simulink model "Dinamica_longitudinale_leader_ubuntu_param"  (R2020b)
settings: Solver=ode23s  StartTime=0.0  StopTime=100  FixedStep=0.0001
model workspace (MAT data in the model file):
  a1 = Simulink.Parameter
  a1.Value = 2
  a1.DataType = 'auto'
  a1.Dimensions = [1 1]
  a2 = Simulink.Parameter
  a2.Value = 0.5
  a2.DataType = 'auto'
  a2.Dimensions = [1 1]
  a3 = Simulink.Parameter
  a3.Value = -1.5
  a3.DataType = 'auto'
  a3.Dimensions = [1 1]
  a4 = Simulink.Parameter
  a4.Value = 1.2
  a4.DataType = 'auto'
  a4.Dimensions = [1 1]
  a5 = Simulink.Parameter
  a5.Value = -1
  a5.DataType = 'auto'
  a5.Dimensions = [1 1]
  a6 = Simulink.Parameter
  a6.Value = 1
  a6.DataType = 'auto'
  a6.Dimensions = [1 1]
  aero_drag_coeff = Simulink.Parameter
  aero_drag_coeff.Value = 0.3
  aero_drag_coeff.DataType = 'auto'
  aero_drag_coeff.Dimensions = [1 1]
  frontal_area = Simulink.Parameter
  frontal_area.Value = 2
  frontal_area.DataType = 'auto'
  frontal_area.Dimensions = [1 1]
  initialDesiredSpeed = Simulink.Parameter
  initialDesiredSpeed.Value = 0
  initialDesiredSpeed.DataType = 'auto'
  initialDesiredSpeed.Dimensions = [1 1]
  initialPosition = Simulink.Parameter
  initialPosition.Value = 10
  initialPosition.DataType = 'auto'
  initialPosition.Dimensions = [1 1]
  initialRotation = Simulink.Parameter
  initialRotation.Value = 0.001
  initialRotation.DataType = 'auto'
  initialRotation.Dimensions = [1 1]
  initialSpeed = Simulink.Parameter
  initialSpeed.Value = 0.001
  initialSpeed.DataType = 'auto'
  initialSpeed.Dimensions = [1 1]
  k = Simulink.Parameter
  k.Value = 500
  k.DataType = 'auto'
  k.Dimensions = [1 1]
  mass = Simulink.Parameter
  mass.Value = 1350
  mass.DataType = 'auto'
  mass.Dimensions = [1 1]
  maxRotation = Simulink.Parameter
  maxRotation.Value = 1000000
  maxRotation.DataType = 'auto'
  maxRotation.Dimensions = [1 1]
  maxSpeed = Simulink.Parameter
  maxSpeed.Value = 50
  maxSpeed.DataType = 'auto'
  maxSpeed.Dimensions = [1 1]
  minRotation = Simulink.Parameter
  minRotation.Value = -1000000
  minRotation.DataType = 'auto'
  minRotation.Dimensions = [1 1]
  minSpeed = Simulink.Parameter
  minSpeed.Value = -50
  minSpeed.DataType = 'auto'
  minSpeed.Dimensions = [1 1]
  t1 = Simulink.Parameter
  t1.Value = 10
  t1.DataType = 'auto'
  t1.Dimensions = [1 1]
  t1_wet = Simulink.Parameter
  t1_wet.Value = 999
  t1_wet.DataType = 'auto'
  t1_wet.Dimensions = [1 1]
  t2 = Simulink.Parameter
  t2.Value = 20
  t2.DataType = 'auto'
  t2.Dimensions = [1 1]
  t2_snow = Simulink.Parameter
  t2_snow.Value = 999
  t2_snow.DataType = 'auto'
  t2_snow.Dimensions = [1 1]
  t3 = Simulink.Parameter
  t3.Value = 30
  t3.DataType = 'auto'
  t3.Dimensions = [1 1]
  t3_ice = Simulink.Parameter
  t3_ice.Value = 999
  t3_ice.DataType = 'auto'
  t3_ice.Dimensions = [1 1]
  t4 = Simulink.Parameter
  t4.Value = 40
  t4.DataType = 'auto'
  t4.Dimensions = [1 1]
  t5 = Simulink.Parameter
  t5.Value = 50
  t5.DataType = 'auto'
  t5.Dimensions = [1 1]
  v_height = Simulink.Parameter
  v_height.Value = 0.75
  v_height.DataType = 'auto'
  v_height.Dimensions = [1 1]
libraries: simulink x1
settings Model: ParameterArgumentNames=a1,a2,a3,a4,a5,a6,aero_drag_coeff,frontal_area,initialDesiredSpeed,initialPosition,initialRotation,initialSpeed,k,mass,maxRotation,maxSpeed,minRotation,minSpeed,t1,t1_wet,t2,t2_snow,t3,t3_ice,t4,t5,v_height  OrderedModelArguments=off  Creator=salvo  LastModifiedBy=ubuntu

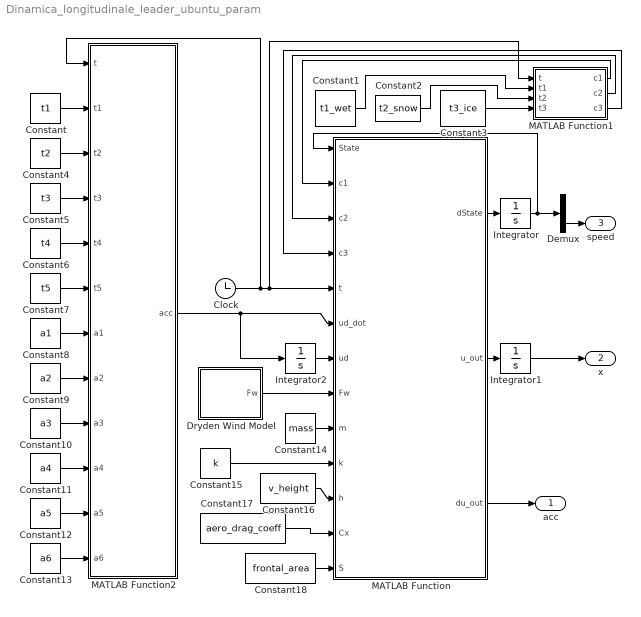
== system Dinamica_longitudinale_leader_ubuntu_param ==
  Clock : Clock
  Constant : Constant  Value=t1
  Constant1 : Constant  Value=t1_wet
  Constant10 : Constant  Value=a3
  Constant11 : Constant  Value=a4
  Constant12 : Constant  Value=a5
  Constant13 : Constant  Value=a6
  Constant14 : Constant  Value=mass
  Constant15 : Constant  Value=k
  Constant16 : Constant  Value=v_height
  Constant17 : Constant  Value=aero_drag_coeff
  Constant18 : Constant  Value=frontal_area
  Constant2 : Constant  Value=t2_snow
  Constant3 : Constant  Value=t3_ice
  Constant4 : Constant  Value=t2
  Constant5 : Constant  Value=t3
  Constant6 : Constant  Value=t4
  Constant7 : Constant  Value=t5
  Constant8 : Constant  Value=a1
  Constant9 : Constant  Value=a2
  Demux : Demux  Outputs=2
  Dryden Wind Model : Subsystem
  Integrator : Integrator  InitialCondition=[initialRotation;initialSpeed]  LimitOutput=on  UpperSaturationLimit=[maxRotation;maxSpeed]  LowerSaturationLimit=[minRotation;minSpeed]
  Integrator1 : Integrator  InitialCondition=initialPosition
  Integrator2 : Integrator  InitialCondition=initialDesiredSpeed  LimitOutput=on  UpperSaturationLimit=maxSpeed  LowerSaturationLimit=minSpeed
  MATLAB Function : MATLAB Function  TreatAsAtomicUnit=on
  MATLAB Function1 : MATLAB Function  TreatAsAtomicUnit=on
  MATLAB Function2 : MATLAB Function  TreatAsAtomicUnit=on
  acc : Outport
  x : Outport  Port=2
  speed : Outport  Port=3
  wires:
  MATLAB Function/1(dState) -> Integrator/1
  Integrator/1 -> Demux/1, MATLAB Function/1(State)
  Clock/1 -> MATLAB Function2/1(t), MATLAB Function1/1(t), MATLAB Function/5(t)
  MATLAB Function2/1(acc) -> MATLAB Function/6(ud_dot), Integrator2/1
  MATLAB Function/2(u_out) -> Integrator1/1
  Integrator1/1 -> x/1
  Integrator2/1 -> MATLAB Function/7(ud)
  MATLAB Function1/3(c3) -> MATLAB Function/4(c3)
  MATLAB Function1/2(c2) -> MATLAB Function/3(c2)
  MATLAB Function1/1(c1) -> MATLAB Function/2(c1)
  MATLAB Function/3(du_out) -> acc/1
  Dryden Wind Model/1(Fw) -> MATLAB Function/8(Fw)
  Demux/2 -> speed/1
  Constant1/1 -> MATLAB Function1/2(t1)
  Constant2/1 -> MATLAB Function1/3(t2)
  Constant3/1 -> MATLAB Function1/4(t3)
  Constant/1 -> MATLAB Function2/2(t1)
  Constant4/1 -> MATLAB Function2/3(t2)
  Constant5/1 -> MATLAB Function2/4(t3)
  Constant13/1 -> MATLAB Function2/12(a6)
  Constant12/1 -> MATLAB Function2/11(a5)
  Constant11/1 -> MATLAB Function2/10(a4)
  Constant6/1 -> MATLAB Function2/5(t4)
  Constant7/1 -> MATLAB Function2/6(t5)
  Constant8/1 -> MATLAB Function2/7(a1)
  Constant9/1 -> MATLAB Function2/8(a2)
  Constant10/1 -> MATLAB Function2/9(a3)
  Constant14/1 -> MATLAB Function/9(m)
  Constant15/1 -> MATLAB Function/10(k)
  Constant16/1 -> MATLAB Function/11(h)
  Constant17/1 -> MATLAB Function/12(Cx)
  Constant18/1 -> MATLAB Function/13(S)

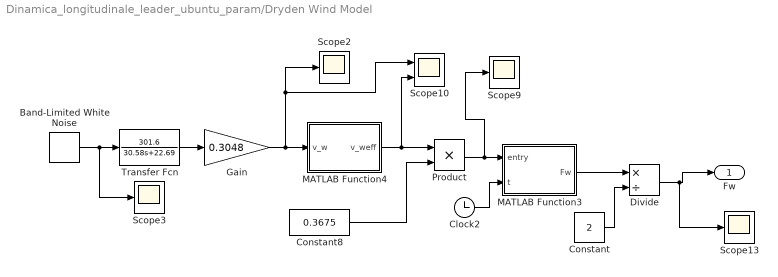
== system Dinamica_longitudinale_leader_ubuntu_param/Dryden Wind Model ==
  Band-Limited White Noise : simulink/Sources/Band-Limited White Noise  Cov=50  Ts=0.1  seed=[23341]
  Clock2 : Clock
  Constant : Constant  Value=2
  Constant8 : Constant  Value=0.3675
  Divide : Product  Inputs=*/
  Gain : Gain  Gain=0.3048
  MATLAB Function3 : MATLAB Function  TreatAsAtomicUnit=on
  MATLAB Function4 : MATLAB Function  TreatAsAtomicUnit=on
  Product : Product
  Scope10 : Scope  NumInputPorts=2
  Scope{2..3,9,13} (4 alike) : Scope
  Transfer Fcn : TransferFcn  Numerator=[301.6]  Denominator=[0 30.58 22.69]
  Fw : Outport  VectorParamsAs1DForOutWhenUnconnected=off
  wires:
  Constant8/1 -> Product/2
  Band-Limited White Noise/1 -> Transfer Fcn/1, Scope3/1
  Product/1 -> Scope9/1, MATLAB Function3/1(entry)
  Clock2/1 -> MATLAB Function3/2(t)
  Gain/1 -> MATLAB Function4/1(v_w), Scope2/1, Scope10/1
  MATLAB Function4/1(v_weff) -> Scope10/2, Product/1
  Transfer Fcn/1 -> Gain/1
  MATLAB Function3/1(Fw) -> Divide/1
  Constant/1 -> Divide/2
  Divide/1 -> Scope13/1, Fw/1

== matlab function Dinamica_longitudinale_leader_ubuntu_param/Dryden Wind Model/MATLAB Function4 ==
  data: v_w input; v_weff output
function v_weff = fcn(v_w)

v_wquadro = (v_w)^2;

if v_w >=0
    v_weff = v_wquadro;
else
    v_weff = -v_wquadro;
end

== matlab function Dinamica_longitudinale_leader_ubuntu_param/MATLAB Function ==
  data: State input; c1 input; c2 input; c3 input; t input; ud_dot input; dState output; ud input; Fw input; u_out output; du_out output; m input; k input; h input; Cx input; S input
function [dState, u_out, du_out] = long_dyn(State, c1, c2, c3, t, ud_dot, ud, Fw, m, k, h, Cx, S) 
%c1,c2 e c3 sono i coefficienti di Burckhardt per il calcolo dell'attrito
%ud --> velocità desiderata
%ud_dot --> accelerazione desiderata (derivata di ud)
%Fw --> Forza del vento opposta al senso di marcia

w = State(1);   % rotazione ruota
u = State(2);   % velocità long

%m = 1350; %Massa del veicolo [Kg]

ro = 1.225; %Densità dell'aria [Kg/m^3]
%S = 2; %Superficie bagnata longitudinale [m^2]
%Cx = 0.3; %Coefficiente di resistenza longitudinale 
F_aero = 0.5*ro*S*Cx*u^2; %Forza aerodinamica [N] - formula 4.2 cap.4

%f = 0.01; %Coefficiente di resistenza al rotolamento
g = 9.81; %Accelerazione di gravità [m/s^2]
a1 = 1.51; %Semipasso anteriore [m]
a2 = 1.288; %Semipasso posteriore [m]
l = a1+a2; %Passo [m]

C0 = 9.91*10^-3; %Coefficienti tipici per pneumatici radiali
C1 = 1.95*10^-5;
C2 = 1.76*10^-9;
Rxt = C0+C1*u+C2*u^4; %Resistenza al rotolamento complessiva [N]

%Fattori contrastanti il senso di marcia - formula 4.1. 
%Include Fw che è il vento
FLoss = Fw+Rxt+F_aero;

Iw = 1.125; % momento inerziale della ruota [Kg*m^2]
%h = 0.75; % Altezza del baricentro rispetto al suolo [m]

FzR = m*g*a1/l + m*h*ud_dot/l; %Trasferimento di carico assale posteriore [N]
Fz = FzR; %Carico normale totale agente sulla vettura [N]
kt = 150000; %Rigidezza verticale ruota motrice [N/m]

R_w = 0.5; %Raggio indeformato [m]
R_s = R_w - Fz/kt; %Raggio statico [m]
x = acos(complex(R_s/R_w));
R = real((sin(x)/x)*R_w); %Raggio effettivo [m]

%k = 500;

%calcolo coppia desiderata (eq.28 paper "Pedone")
Tw = (Iw/R)*(ud_dot - k*(u-ud));

if w*R>u
    sigma = (w*R-u)/(w*R); %Slittamento longitudinale in fase di accelerazione 
elseif (w*R)==u
    sigma = 0;
else
    sigma = (w*R-u)/u; %Slittamento longitudinale in fase di frenatura
end

mu = c1*(1-exp(-c2*sigma))-c3*sigma;

% Forza longitudinale delle ruote (Fxf+Fxr)
Fx2 = mu*Fz; 

dw = 1/Iw*(Tw-R*Fx2); %Dinamica rotazionale ruota motrice - (4.38)
du = 1/m*(Fx2-FLoss); %Din Longitudinale - (4.1)

dState = [dw du]';
u_out = u;

if t<0.1
    du_out = 0;
else
    du_out = du;
end

end

== matlab function Dinamica_longitudinale_leader_ubuntu_param/MATLAB Function2 ==
  data: t input; acc output; t1 input; t2 input; t3 input; t4 input; t5 input; a1 input; a2 input; a3 input; a4 input; a5 input; a6 input
function acc  = driver_acc(t, t1, t2, t3, t4, t5, a1, a2, a3, a4, a5, a6)

if t < t1
    acc = a1;
elseif t < t2
    acc = a2;
elseif t < t3
    acc = a3;
elseif t < t4
    acc = a4;
elseif t < t5
    acc = a5;
else
    acc = a6;
end

== matlab function Dinamica_longitudinale_leader_ubuntu_param/MATLAB Function1 ==
  data: t input; c1 output; c2 output; c3 output; t1 input; t2 input; t3 input
function [c1, c2, c3] = fcn(t, t1, t2, t3)

Burckhardt = [...
    1.29, 23.99, 0.52; ... % dry
    0.86, 33.82, 0.35; ... % wet
    0.19, 94.13, 0.05; ... % snow
    0.05, 306.39, 0];      % ice

if t < t1
    c = Burckhardt(1,:);
elseif t < t2
    c = Burckhardt(2,:);
elseif t < t3
    c = Burckhardt(3,:);
else
    c = Burckhardt(4,:);
end

c1 = c(1);
c2 = c(2);
c3 = c(3);

== matlab function Dinamica_longitudinale_leader_ubuntu_param/Dryden Wind Model/MATLAB Function3 ==
  data: entry input; Fw output; t input
function Fw = fcn(entry,t)

if t<2
    Fw = 0;
else
    Fw = entry;
end
